simulink model "ase_augmented_state_estimator_hrn"  (R2015b)
settings: Solver=FixedStepDiscrete  StartTime=0.0  StopTime=test_stop_time  FixedStep=astrobee_time_step_size  RelTol=1e-3
values from neighbouring files (symbols this model uses):
  cvs_registration_pulse_IC = Simulink.Bus.createMATLABStruct('cvs_registration_pulse')    [ase_hw_data_test.m]
  numOF_pts = 50    [ase_hw_data_test.m]
undefined symbols (not defined in the file or in its folder): astrobee_time_step_size, bus_cmc_msg_ic, cvs_handrail_pulse, cvs_landmark_pulse, cvs_optical_flow_pulse, localization_mode_cmd, speed_gain_cmd
libraries: est_estimator_lib_wState_lib x1
settings Model: Creator=jfusco1  LastModifiedBy=jfusco1
settings DataIOCC: SaveFormat=Array
settings HardwareCC: ProdBitPerPointer=32  ProdLargestAtomicFloat=None  ProdIntDivRoundTo=Undefined  ProdEndianess=Unspecified  ProdWordSize=32  ProdHWDeviceType=32-bit Generic
settings GRTTargetCC: GeneratePreprocessorConditionals=Disable all
settings ConfigComp: CovModelRefEnable=Off

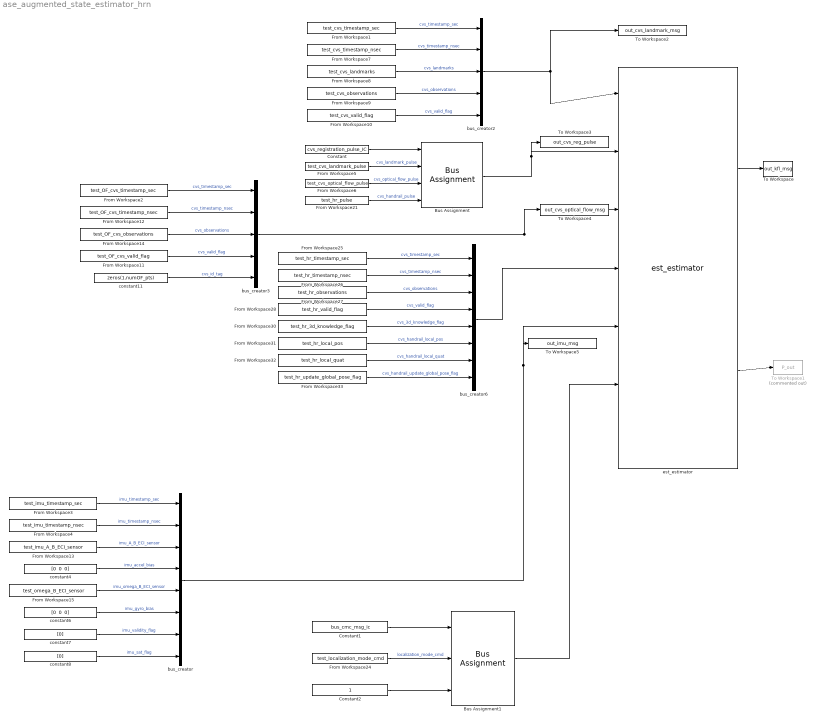
== system ase_augmented_state_estimator_hrn ==
  Bus Assignment : BusAssignment  AssignedSignals=cvs_landmark_pulse,cvs_optical_flow_pulse,cvs_handrail_pulse
  Bus Assignment1 : BusAssignment  AssignedSignals=localization_mode_cmd,speed_gain_cmd
  Constant : Constant  Value=cvs_registration_pulse_IC  OutDataTypeStr=Bus: cvs_registration_pulse
  Constant1 : Constant  Value=bus_cmc_msg_ic  OutDataTypeStr=Bus: cmc_msg
  Constant2 : Constant  OutDataTypeStr=uint8
  From Workspace1 : FromWorkspace  VariableName=test_cvs_timestamp_sec  SampleTime=0  Interpolate=off  OutputAfterFinalValue=Holding final value
  From Workspace10 : FromWorkspace  VariableName=test_cvs_valid_flag  SampleTime=0  Interpolate=off  OutputAfterFinalValue=Holding final value
  From Workspace11 : FromWorkspace  VariableName=test_OF_cvs_valid_flag  SampleTime=0  Interpolate=off  OutputAfterFinalValue=Holding final value
  From Workspace12 : FromWorkspace  VariableName=test_OF_cvs_timestamp_nsec  SampleTime=0  Interpolate=off  OutputAfterFinalValue=Holding final value
  From Workspace13 : FromWorkspace  VariableName=test_imu_A_B_ECI_sensor  SampleTime=0  Interpolate=off  OutputAfterFinalValue=Holding final value
  From Workspace14 : FromWorkspace  VariableName=test_OF_cvs_observations  SampleTime=0  Interpolate=off  OutputAfterFinalValue=Holding final value
  From Workspace15 : FromWorkspace  VariableName=test_omega_B_ECI_sensor  SampleTime=0  Interpolate=off  OutputAfterFinalValue=Holding final value
  From Workspace2 : FromWorkspace  VariableName=test_OF_cvs_timestamp_sec  SampleTime=0  Interpolate=off  OutputAfterFinalValue=Holding final value
  From Workspace21 : FromWorkspace  VariableName=test_hr_pulse  SampleTime=0  Interpolate=off  OutputAfterFinalValue=Holding final value
  From Workspace24 : FromWorkspace  VariableName=test_localization_mode_cmd  SampleTime=0  Interpolate=off  OutputAfterFinalValue=Holding final value
  From Workspace25 : FromWorkspace  VariableName=test_hr_timestamp_sec  SampleTime=astrobee_time_step_size  Interpolate=off  OutputAfterFinalValue=Holding final value
  From Workspace26 : FromWorkspace  VariableName=test_hr_timestamp_nsec  SampleTime=astrobee_time_step_size  Interpolate=off  OutputAfterFinalValue=Holding final value
  From Workspace27 : FromWorkspace  VariableName=test_hr_observations  SampleTime=astrobee_time_step_size  Interpolate=off  OutputAfterFinalValue=Holding final value
  From Workspace28 : FromWorkspace  VariableName=test_hr_valid_flag  SampleTime=astrobee_time_step_size  Interpolate=off  OutputAfterFinalValue=Holding final value
  From Workspace3 : FromWorkspace  VariableName=test_imu_timestamp_sec  SampleTime=0  Interpolate=off  OutputAfterFinalValue=Holding final value
  From Workspace30 : FromWorkspace  VariableName=test_hr_3d_knowledge_flag  SampleTime=astrobee_time_step_size  Interpolate=off  OutputAfterFinalValue=Holding final value
  From Workspace31 : FromWorkspace  VariableName=test_hr_local_pos  SampleTime=astrobee_time_step_size  Interpolate=off  OutputAfterFinalValue=Holding final value
  From Workspace32 : FromWorkspace  VariableName=test_hr_local_quat  SampleTime=astrobee_time_step_size  Interpolate=off  OutputAfterFinalValue=Holding final value
  From Workspace33 : FromWorkspace  VariableName=test_hr_update_global_pose_flag  SampleTime=astrobee_time_step_size  Interpolate=off  OutputAfterFinalValue=Holding final value
  From Workspace4 : FromWorkspace  VariableName=test_imu_timestamp_nsec  SampleTime=0  Interpolate=off  OutputAfterFinalValue=Holding final value
  From Workspace5 : FromWorkspace  VariableName=test_cvs_landmark_pulse  SampleTime=0  Interpolate=off  OutputAfterFinalValue=Holding final value
  From Workspace6 : FromWorkspace  VariableName=test_cvs_optical_flow_pulse  SampleTime=0  Interpolate=off  OutputAfterFinalValue=Holding final value
  From Workspace7 : FromWorkspace  VariableName=test_cvs_timestamp_nsec  SampleTime=0  Interpolate=off  OutputAfterFinalValue=Holding final value
  From Workspace8 : FromWorkspace  VariableName=test_cvs_landmarks  SampleTime=0  Interpolate=off  OutputAfterFinalValue=Holding final value
  From Workspace9 : FromWorkspace  VariableName=test_cvs_observations  SampleTime=0  Interpolate=off  OutputAfterFinalValue=Holding final value
  To Workspace : ToWorkspace  VariableName=out_kfl_msg  SaveFormat=Timeseries  SampleTime=-1
  To Workspace1 : ToWorkspace  Commented=on  VariableName=P_out  SaveFormat=Timeseries  SampleTime=-1
  To Workspace2 : ToWorkspace  VariableName=out_cvs_landmark_msg  SaveFormat=Timeseries  SampleTime=-1
  To Workspace3 : ToWorkspace  VariableName=out_cvs_reg_pulse  SaveFormat=Timeseries  SampleTime=-1
  To Workspace4 : ToWorkspace  VariableName=out_cvs_optical_flow_msg  SaveFormat=Timeseries  SampleTime=-1
  To Workspace5 : ToWorkspace  VariableName=out_imu_msg  SaveFormat=Timeseries  SampleTime=-1
  bus_creator : BusCreator  Inputs=8
  bus_creator2 : BusCreator  Inputs=5
  bus_creator3 : BusCreator  Inputs=5
  bus_creator6 : BusCreator  Inputs=8
  constant11 : Constant  Value=zeros(1,numOF_pts)  OutDataTypeStr=single
  constant4 : Constant  Value="[0  0  0]"  OutDataTypeStr=single
  constant6 : Constant  Value="[0  0  0]"  OutDataTypeStr=single
  constant7 : Constant  Value=[0]  OutDataTypeStr=uint8
  constant8 : Constant  Value=[0]  OutDataTypeStr=uint8
  est_estimator : est_estimator_lib_wState_lib/est_estimator
  wires:
  bus_creator2/1 -> To Workspace2/1, est_estimator/1
  bus_creator3/1 -> To Workspace4/1, est_estimator/3
  est_estimator/1 -> To Workspace/1
  est_estimator/2 -> To Workspace1/1
  From Workspace3/1 -> bus_creator/1  "imu_timestamp_sec"
  From Workspace4/1 -> bus_creator/2  "imu_timestamp_nsec"
  From Workspace13/1 -> bus_creator/3  "imu_A_B_ECI_sensor"
  constant4/1 -> bus_creator/4  "imu_accel_bias"
  From Workspace15/1 -> bus_creator/5  "imu_omega_B_ECI_sensor"
  constant6/1 -> bus_creator/6  "imu_gyro_bias"
  constant7/1 -> bus_creator/7  "imu_validity_flag"
  constant8/1 -> bus_creator/8  "imu_sat_flag"
  From Workspace1/1 -> bus_creator2/1  "cvs_timestamp_sec"
  From Workspace7/1 -> bus_creator2/2  "cvs_timestamp_nsec"
  From Workspace8/1 -> bus_creator2/3  "cvs_landmarks"
  From Workspace9/1 -> bus_creator2/4  "cvs_observations"
  From Workspace10/1 -> bus_creator2/5  "cvs_valid_flag"
  From Workspace2/1 -> bus_creator3/1  "cvs_timestamp_sec"
  From Workspace12/1 -> bus_creator3/2  "cvs_timestamp_nsec"
  From Workspace14/1 -> bus_creator3/3  "cvs_observations"
  From Workspace11/1 -> bus_creator3/4  "cvs_valid_flag"
  constant11/1 -> bus_creator3/5  "cvs_id_tag"
  bus_creator/1 -> est_estimator/5, To Workspace5/1
  Bus Assignment1/1 -> est_estimator/6
  From Workspace25/1 -> bus_creator6/1  "cvs_timestamp_sec"
  From Workspace26/1 -> bus_creator6/2  "cvs_timestamp_nsec"
  From Workspace27/1 -> bus_creator6/3  "cvs_observations"
  From Workspace28/1 -> bus_creator6/4  "cvs_valid_flag"
  From Workspace30/1 -> bus_creator6/5  "cvs_3d_knowledge_flag"
  bus_creator6/1 -> est_estimator/4
  From Workspace31/1 -> bus_creator6/6  "cvs_handrail_local_pos"
  From Workspace32/1 -> bus_creator6/7  "cvs_handrail_local_quat"
  From Workspace33/1 -> bus_creator6/8  "cvs_handrail_update_global_pose_flag"
  Constant/1 -> Bus Assignment/1
  From Workspace6/1 -> Bus Assignment/3  "cvs_optical_flow_pulse"
  From Workspace21/1 -> Bus Assignment/4  "cvs_handrail_pulse"
  From Workspace5/1 -> Bus Assignment/2  "cvs_landmark_pulse"
  Bus Assignment/1 -> To Workspace3/1, est_estimator/2
  Constant1/1 -> Bus Assignment1/1
  From Workspace24/1 -> Bus Assignment1/2  "localization_mode_cmd"
  Constant2/1 -> Bus Assignment1/3
